simulink model "Model_IPS1"  (R2016a)
settings: Solver=ode45  StartTime=0.0  StopTime=1.5
values from neighbouring files (symbols this model uses):
  Imrn = 7.4    [parametriAM.m]
  In = 12.7    [parametriAM.m]
  Ismax = In*sqrt(2)    [parametriAM.m]
  J = 0.019    [parametriAM.m]
  Lm = 0.0493    [parametriAM.m]
  Lr = 0.05315    [parametriAM.m]
  Ls = 0.05315    [parametriAM.m]
  Ls_oc = Ls    (= 0.05315)    [parametriAM.m]
  Lst = sigma*Ls    (= 0.00742111947319)    [parametriAM.m]
  pp = 3    [parametriAM.m]
  Rs = 0.594    [parametriAM.m]
  Rs_oc = Rs    (= 0.594)    [parametriAM.m]
  sigma = 1 - 1/((1+sigmaR)*(1+sigmaS))    (= 0.13962595434)    [parametriAM.m]
  sigma_oc = 1 - 1/((1+sigmaR_oc)*(1+sigmaS_oc))    (= 0.13962595434)    [parametriAM.m]
  Tr = Lr/Rr    (= 0.0771407837446)    [parametriAM.m]
  Udc = Un*sqrt(2)    [parametriAM.m]
  Un = 216    [parametriAM.m]
  Usmax = Udc    [parametriAM.m]
libraries: simulink x6
settings Model: Creator=Vaje  LastModifiedBy=Mitja1

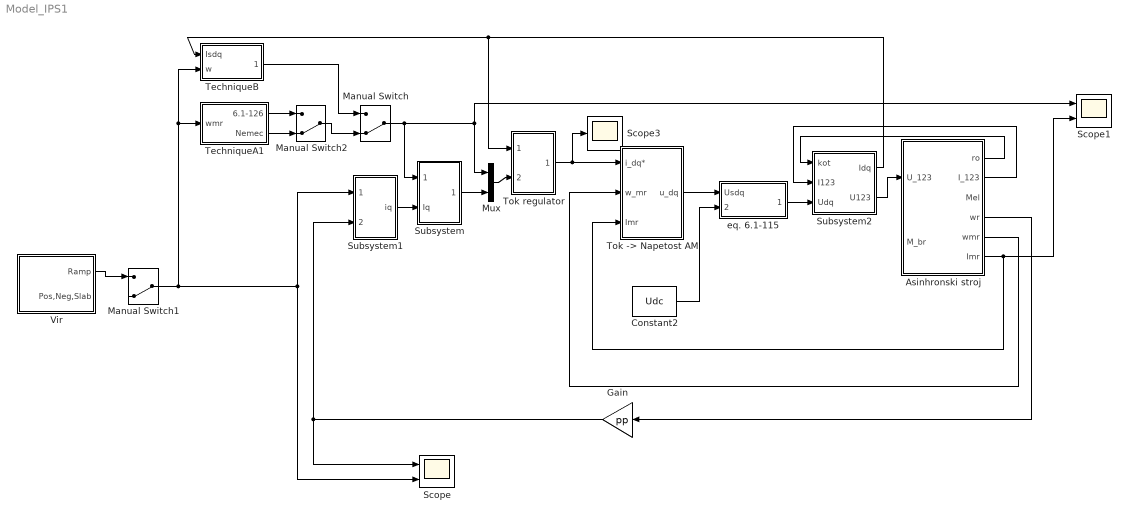
== system Model_IPS1 ==
  Asinhronski stroj : Subsystem  InitFcn=parametriAM
  Constant2 : Constant  Value=Udc
  Gain : Gain  Gain=pp
  Manual Switch : ManualSwitch  CurrentSetting=0
  Manual Switch1 : ManualSwitch  CurrentSetting=0
  Manual Switch2 : ManualSwitch  CurrentSetting=0
  Mux : Mux  Inputs=2
  Scope : Scope  NumInputPorts=2
  Scope1 : Scope  NumInputPorts=2
  Scope3 : Scope
  Subsystem : Subsystem
  Subsystem1 : Subsystem
  Subsystem2 : Subsystem
  TechniqueA1 : Subsystem
  TechniqueB : Subsystem
  "Tok -> Napetost AM" : Subsystem
  Tok regulator : Subsystem
  Vir : Subsystem
  eq. 6.1-115 : Subsystem
  wires:
  Constant2/1 -> eq. 6.1-115/2(Usmax)
  "Tok -> Napetost AM"/1(u_dq) -> eq. 6.1-115/1(Usdq)
  Asinhronski stroj/6(Imr) -> Scope1/2, "Tok -> Napetost AM"/3(Imr)
  Asinhronski stroj/5(wmr) -> "Tok -> Napetost AM"/2(w_mr)
  Tok regulator/1(Idq) -> Scope3/1, "Tok -> Napetost AM"/1(i_dq*)
  Gain/1 -> Scope/1, Subsystem1/2(wfdb)
  Subsystem1/1(iq) -> Subsystem/2(Iq)
  Asinhronski stroj/4(wr) -> Gain/1
  Manual Switch/1 -> Subsystem/1(Idref), Mux/1, Scope1/1
  Manual Switch1/1 -> TechniqueB/2(w), TechniqueA1/1(wmr), Subsystem1/1(wref), Scope/2
  Subsystem/1(Iqlim) -> Mux/2
  TechniqueA1/1(6.1-126) -> Manual Switch2/1
  TechniqueA1/2(Nemec) -> Manual Switch2/2
  Vir/1(Ramp) -> Manual Switch1/1
  Subsystem2/1(Idq) -> Tok regulator/1(Idqdej), TechniqueB/1(Isdq)
  Asinhronski stroj/1(ro) -> Subsystem2/1(kot)
  Asinhronski stroj/2(I_123) -> Subsystem2/2(I123)
  eq. 6.1-115/1(Usdqlim) -> Subsystem2/3(Udq)
  Subsystem2/2(U123) -> Asinhronski stroj/1(U_123)
  TechniqueB/1(6.1-135) -> Manual Switch/1
  Manual Switch2/1 -> Manual Switch/2
  Mux/1 -> Tok regulator/2(Idqref)

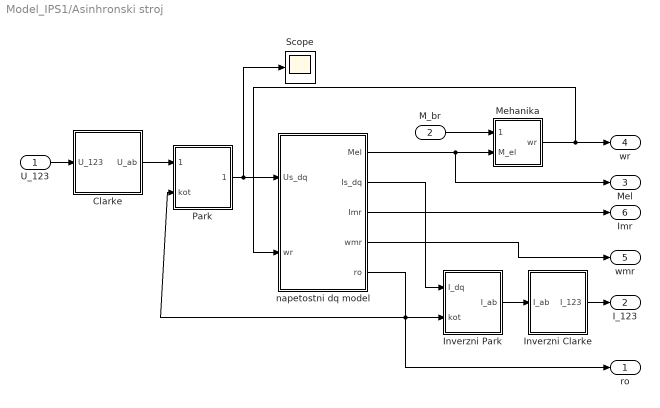
== system Model_IPS1/Asinhronski stroj ==
  U_123 : Inport
  M_br : Inport  Port=2
  Clarke : Subsystem
  Inverzni Clarke : Subsystem
  Inverzni Park : Subsystem
  Mehanika : Subsystem
  Park : Subsystem
  Scope : Scope
  napetostni dq model : Subsystem
  ro : Outport
  I_123 : Outport  Port=2
  Mel : Outport  Port=3
  wr : Outport  Port=4
  wmr : Outport  Port=5
  Imr : Outport  Port=6
  wires:
  Inverzni Park/1(I_ab) -> Inverzni Clarke/1(I_ab)
  Clarke/1(U_ab) -> Park/1(U_ab)
  Mehanika/1(wr) -> napetostni dq model/2(wr), wr/1
  M_br/1 -> Mehanika/1(M_br)
  napetostni dq model/1(Mel) -> Mel/1, Mehanika/2(M_el)
  Inverzni Clarke/1(I_123) -> I_123/1
  napetostni dq model/4(wmr) -> wmr/1
  napetostni dq model/3(Imr) -> Imr/1
  U_123/1 -> Clarke/1(U_123)
  napetostni dq model/2(Is_dq) -> Inverzni Park/1(I_dq)
  napetostni dq model/5(ro) -> ro/1, Park/2(kot), Inverzni Park/2(kot)
  Park/1(U_dq) -> Scope/1, napetostni dq model/1(Us_dq)

== system Model_IPS1/Subsystem ==
  Idref : Inport
  Iq : Inport  Port=2
  Add1 : Sum  Inputs=-+
  Constant : Constant  Value=In*sqrt(2)
  Gain1 : Gain  Gain=-1
  Product : Product
  Product1 : Product
  Saturation Dynamic : simulink/Discontinuities/Saturation Dynamic  OutMin=[]  OutMax=[]  OutDataTypeStr=Inherit: Same as second input  OutDataType=fixdt(1, 16)  OutScaling=2^-10  DoSatur=off
  Sqrt : Sqrt  SaturateOnIntegerOverflow=on
  Iqlim : Outport
  wires:
  Constant/1 -> Product/1, Product/2
  Sqrt/1 -> Gain1/1, Saturation Dynamic/1
  Product1/1 -> Add1/1
  Gain1/1 -> Saturation Dynamic/3
  Add1/1 -> Sqrt/1
  Iq/1 -> Saturation Dynamic/2
  Idref/1 -> Product1/2, Product1/1
  Saturation Dynamic/1 -> Iqlim/1
  Product/1 -> Add1/2

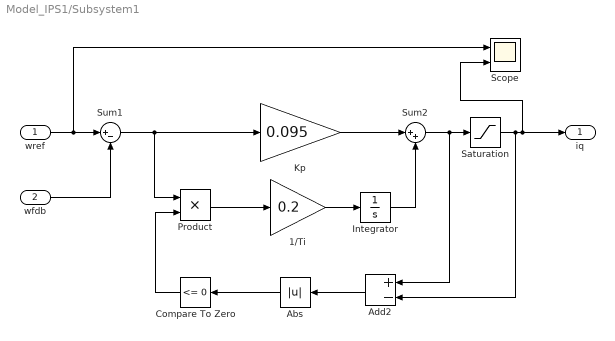
== system Model_IPS1/Subsystem1 ==
  wref : Inport
  wfdb : Inport  Port=2
  1/Ti : Gain  Gain=0.2  SaturateOnIntegerOverflow=on  OutDataTypeStr=Inherit: Same as input  ParamDataTypeStr=Inherit: Same as input
  Abs : Abs
  Add2 : Sum  Inputs=+-
  Compare To Zero : simulink/Logic and Bit Operations/Compare To Zero  relop=<=  OutDataTypeStr=boolean
  Integrator : Integrator
  Kp : Gain  Gain=0.095  SaturateOnIntegerOverflow=on  OutDataTypeStr=Inherit: Same as input  ParamDataTypeStr=Inherit: Same as input
  Product : Product
  Saturation : Saturate  UpperLimit=In*3  LowerLimit=-3*In
  Scope : Scope  NumInputPorts=2
  Sum1 : Sum  Inputs=|+-
  Sum2 : Sum  Inputs=|++
  iq : Outport
  wires:
  1/Ti/1 -> Integrator/1
  Sum1/1 -> Product/1, Kp/1
  Integrator/1 -> Sum2/2
  Sum2/1 -> Add2/1, Saturation/1
  Add2/1 -> Abs/1
  Saturation/1 -> Add2/2, Scope/2, iq/1
  Abs/1 -> Compare To Zero/1
  Kp/1 -> Sum2/1
  Compare To Zero/1 -> Product/2
  Product/1 -> 1/Ti/1
  wref/1 -> Scope/1, Sum1/1
  wfdb/1 -> Sum1/2

== system Model_IPS1/Subsystem2 ==
  kot : Inport
  I123 : Inport  Port=2
  Udq : Inport  Port=3
  Clarke : Subsystem
  Inverzni Clarke : Subsystem
  Inverzni Park : Subsystem
  Park : Subsystem
  Idq : Outport
  U123 : Outport  Port=2
  wires:
  Inverzni Clarke/1(U_123) -> U123/1
  Park/1(I_dq) -> Idq/1
  kot/1 -> Park/2(kot), Inverzni Park/1(kot)
  Clarke/1(I_ab) -> Park/1(I_ab)
  Inverzni Park/1(U_ab) -> Inverzni Clarke/1(U_ab)
  Udq/1 -> Inverzni Park/2(U_dq)
  I123/1 -> Clarke/1(I_123)

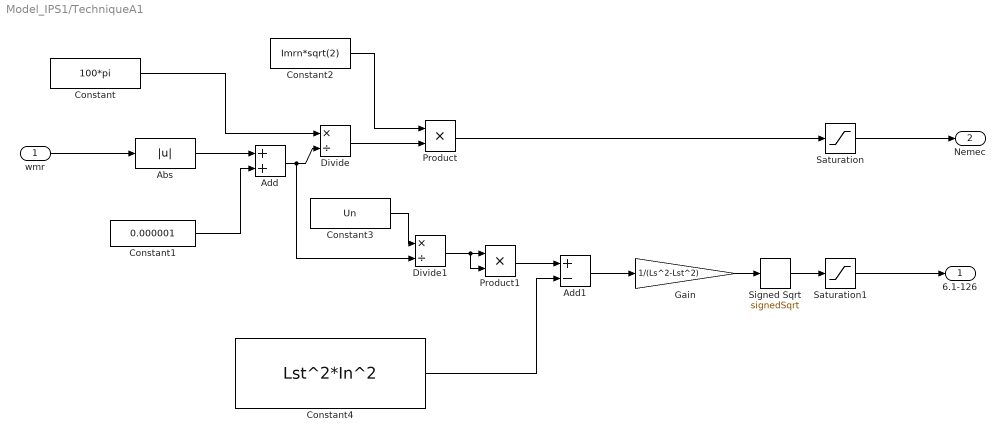
== system Model_IPS1/TechniqueA1 ==
  wmr : Inport
  Abs : Abs
  Add : Sum
  Add1 : Sum  Inputs=+-
  Constant : Constant  Value=100*pi
  Constant1 : Constant  Value=0.000001
  Constant2 : Constant  Value=Imrn*sqrt(2)
  Constant3 : Constant  Value=Un
  Constant4 : Constant  Value=Lst^2*In^2
  Divide : Product  Inputs=*/
  Divide1 : Product  Inputs=*/
  Gain : Gain  Gain=1/(Ls^2-Lst^2)
  Product : Product
  Product1 : Product
  Saturation : Saturate  UpperLimit=+Imrn*sqrt(2)  LowerLimit=0
  Saturation1 : Saturate  UpperLimit=+Imrn*sqrt(2)  LowerLimit=0
  Signed Sqrt : Sqrt  Operator=signedSqrt  SaturateOnIntegerOverflow=on
  6.1-126 : Outport
  Nemec : Outport  Port=2
  wires:
  Constant2/1 -> Product/1
  wmr/1 -> Abs/1
  Divide/1 -> Product/2
  Product/1 -> Saturation/1
  Constant/1 -> Divide/1
  Add/1 -> Divide1/2, Divide/2
  Abs/1 -> Add/1
  Constant1/1 -> Add/2
  Saturation/1 -> Nemec/1
  Constant3/1 -> Divide1/1
  Divide1/1 -> Product1/2, Product1/1
  Product1/1 -> Add1/1
  Constant4/1 -> Add1/2
  Saturation1/1 -> 6.1-126/1
  Add1/1 -> Gain/1
  Gain/1 -> Signed Sqrt/1
  Signed Sqrt/1 -> Saturation1/1

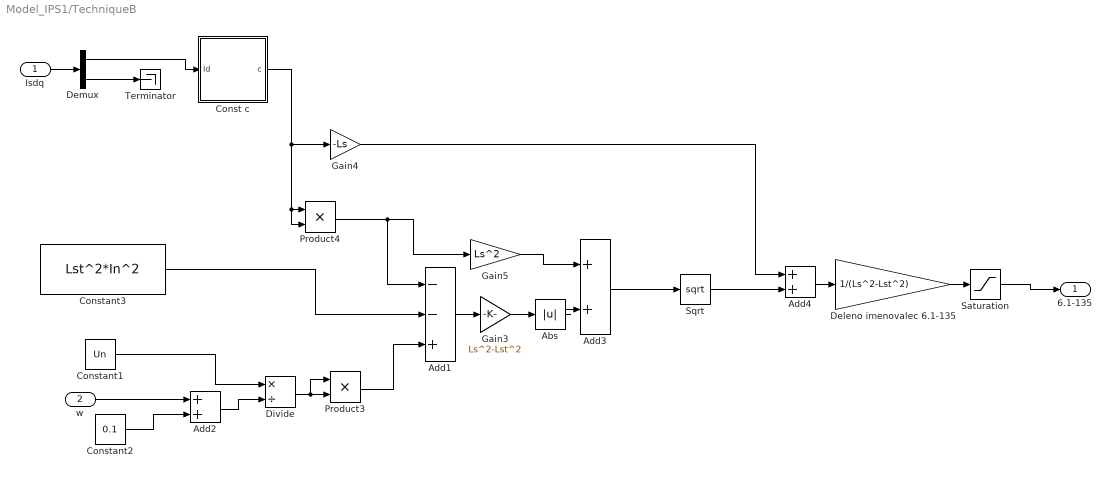
== system Model_IPS1/TechniqueB ==
  Isdq : Inport
  w : Inport  Port=2
  Abs : Abs
  Add1 : Sum  Inputs=--+
  Add2 : Sum
  Add3 : Sum
  Add4 : Sum
  Const c : Subsystem
  Constant1 : Constant  Value=Un
  Constant2 : Constant  Value=0.1
  Constant3 : Constant  Value=Lst^2*In^2
  Deleno imenovalec 6.1-135 : Gain  Gain=1/(Ls^2-Lst^2)
  Demux : Demux  Outputs=2
  Divide : Product  Inputs=*/
  Gain3 : Gain  Gain=Ls^2-Lst^2
  Gain4 : Gain  Gain=-Ls
  Gain5 : Gain  Gain=Ls^2
  Product3 : Product
  Product4 : Product
  Saturation : Saturate  UpperLimit=+Imrn*sqrt(2)  LowerLimit=0
  Sqrt : Sqrt  SaturateOnIntegerOverflow=on
  Terminator : Terminator
  6.1-135 : Outport
  wires:
  Isdq/1 -> Demux/1
  Constant1/1 -> Divide/1
  w/1 -> Add2/1
  Constant2/1 -> Add2/2
  Demux/1 -> Const c/1(Id)
  Demux/2 -> Terminator/1
  Saturation/1 -> 6.1-135/1
  Const c/1(c) -> Product4/2, Product4/1, Gain4/1
  Product4/1 -> Add1/1, Gain5/1
  Gain5/1 -> Add3/1
  Gain4/1 -> Add4/1
  Add4/1 -> Deleno imenovalec 6.1-135/1
  Deleno imenovalec 6.1-135/1 -> Saturation/1
  Add1/1 -> Gain3/1
  Constant3/1 -> Add1/2
  Add2/1 -> Divide/2
  Divide/1 -> Product3/1, Product3/2
  Product3/1 -> Add1/3
  Sqrt/1 -> Add4/2
  Gain3/1 -> Abs/1
  Add3/1 -> Sqrt/1
  Abs/1 -> Add3/2

== system Model_IPS1/Tok -> Napetost AM ==
  i_dq* : Inport
  w_mr : Inport  Port=2
  Imr : Inport  Port=3
  Mux : Mux  Inputs=2
  eq 5.146 : Subsystem
  eq 5.147 : Subsystem
  u_dq : Outport
  wires:
  i_dq*/1 -> eq 5.147/1(I_dq), eq 5.146/1(I_dq)
  Mux/1 -> u_dq/1
  w_mr/1 -> eq 5.147/2(w_mr), eq 5.146/2(w_mr)
  Imr/1 -> eq 5.146/3(Imr), eq 5.147/3(Imr)
  eq 5.147/1(u_q) -> Mux/2
  eq 5.146/1(u_d) -> Mux/1

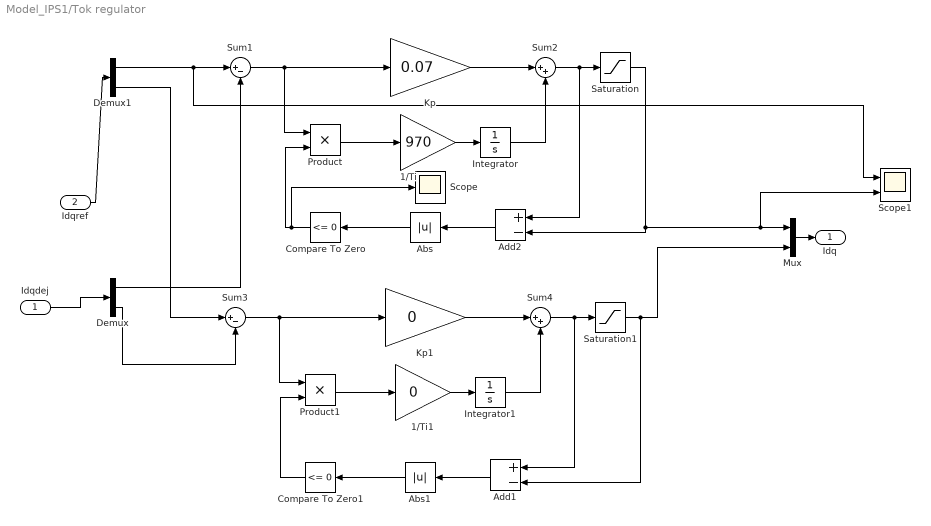
== system Model_IPS1/Tok regulator ==
  Idqdej : Inport
  Idqref : Inport  Port=2
  1/Ti : Gain  Gain=970  SaturateOnIntegerOverflow=on  OutDataTypeStr=Inherit: Same as input  ParamDataTypeStr=Inherit: Same as input
  1/Ti1 : Gain  Gain=0  SaturateOnIntegerOverflow=on  OutDataTypeStr=Inherit: Same as input  ParamDataTypeStr=Inherit: Same as input
  Abs : Abs  ZeroCross=off
  Abs1 : Abs
  Add1 : Sum  Inputs=+-
  Add2 : Sum  Inputs=+-
  Compare To Zero : simulink/Logic and Bit Operations/Compare To Zero  relop=<=  OutDataTypeStr=boolean  ZeroCross=off
  Compare To Zero1 : simulink/Logic and Bit Operations/Compare To Zero  relop=<=  OutDataTypeStr=boolean
  Demux : Demux  Outputs=2
  Demux1 : Demux  Outputs=2
  Integrator : Integrator
  Integrator1 : Integrator
  Kp : Gain  Gain=0.07  SaturateOnIntegerOverflow=on  OutDataTypeStr=Inherit: Same as input  ParamDataTypeStr=Inherit: Same as input
  Kp1 : Gain  Gain=0  SaturateOnIntegerOverflow=on  OutDataTypeStr=Inherit: Same as input  ParamDataTypeStr=Inherit: Same as input
  Mux : Mux  Inputs=2
  Product : Product
  Product1 : Product
  Saturation : Saturate  UpperLimit=Ismax  LowerLimit=-Ismax  ZeroCross=off
  Saturation1 : Saturate  UpperLimit=3*In  LowerLimit=-3*In
  Scope : Scope
  Scope1 : Scope  NumInputPorts=2
  Sum1 : Sum  Inputs=|+-
  Sum2 : Sum  Inputs=|++
  Sum3 : Sum  Inputs=|+-
  Sum4 : Sum  Inputs=|++
  Idq : Outport
  wires:
  Abs1/1 -> Compare To Zero1/1
  Add1/1 -> Abs1/1
  Compare To Zero1/1 -> Product1/2
  Product1/1 -> 1/Ti1/1
  Integrator1/1 -> Sum4/2
  Sum4/1 -> Saturation1/1, Add1/1
  Saturation1/1 -> Mux/2, Add1/2
  Kp1/1 -> Sum4/1
  1/Ti1/1 -> Integrator1/1
  Sum3/1 -> Kp1/1, Product1/1
  Demux1/2 -> Sum3/1
  Idqref/1 -> Demux1/1
  Mux/1 -> Idq/1
  Sum1/1 -> Product/1, Kp/1
  Integrator/1 -> Sum2/2
  Saturation/1 -> Scope1/2, Mux/1, Add2/2
  Kp/1 -> Sum2/1
  Demux1/1 -> Scope1/1, Sum1/1
  1/Ti/1 -> Integrator/1
  Add2/1 -> Abs/1
  Abs/1 -> Compare To Zero/1
  Compare To Zero/1 -> Scope/1, Product/2
  Sum2/1 -> Add2/1, Saturation/1
  Product/1 -> 1/Ti/1
  Idqdej/1 -> Demux/1
  Demux/2 -> Sum3/2
  Demux/1 -> Sum1/2

== system Model_IPS1/Vir ==
  Add1 : Sum  Inputs=++++
  Rampa : simulink/Sources/Ramp  slope=200*pi  start=0  X0=0
  Step : Step  After=100*pi  SampleTime=0
  Step1 : Step  Time=3  After=100*pi  SampleTime=0
  Step2 : Step  Time=5  After=-300*pi  SampleTime=0
  Step3 : Step  Time=7  After=-100*pi  SampleTime=0
  Ramp : Outport
  Pos,Neg,Slab : Outport  Port=2
  wires:
  Add1/1 -> Pos,Neg,Slab/1
  Step1/1 -> Add1/2
  Step2/1 -> Add1/3
  Step/1 -> Add1/1
  Rampa/1 -> Ramp/1
  Step3/1 -> Add1/4

== system Model_IPS1/eq. 6.1-115 ==
  Usdq : Inport
  Usmax : Inport  Port=2
  Demux : Demux  Outputs=2
  Mux1 : Mux  Inputs=2
  eq. 6.1-120 : Subsystem
  Usdqlim : Outport
  wires:
  Mux1/1 -> Usdqlim/1
  Usdq/1 -> Demux/1
  Usmax/1 -> eq. 6.1-120/3(Usmax)
  Demux/2 -> eq. 6.1-120/2(Usq)
  Demux/1 -> eq. 6.1-120/1(Usd), Mux1/1
  eq. 6.1-120/1(Usqlim) -> Mux1/2

== system Model_IPS1/Asinhronski stroj/Clarke ==
  U_123 : Inport
  ABC_ab1 : Subsystem
  Demux : Demux  Outputs=3
  Mux : Mux  Inputs=2
  U_ab : Outport
  wires:
  Mux/1 -> U_ab/1
  ABC_ab1/2(beta) -> Mux/2
  ABC_ab1/1(alfa) -> Mux/1
  Demux/3 -> ABC_ab1/3(C)
  Demux/2 -> ABC_ab1/2(B)
  Demux/1 -> ABC_ab1/1(A)
  U_123/1 -> Demux/1

== system Model_IPS1/Asinhronski stroj/Inverzni Clarke ==
  I_ab : Inport
  Demux : Demux  Outputs=2
  Mux : Mux  Inputs=3
  ab_ABC : Subsystem
  I_123 : Outport
  wires:
  ab_ABC/3(C) -> Mux/3
  ab_ABC/2(B) -> Mux/2
  ab_ABC/1(A) -> Mux/1
  Demux/2 -> ab_ABC/2(beta)
  Demux/1 -> ab_ABC/1(alfa)
  I_ab/1 -> Demux/1
  Mux/1 -> I_123/1

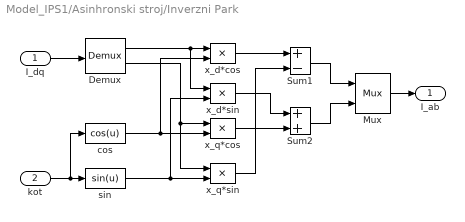
== system Model_IPS1/Asinhronski stroj/Inverzni Park ==
  I_dq : Inport
  kot : Inport  Port=2
  Demux : Demux  Outputs=2
  Mux : Mux  Inputs=2
  "Sum1 " : Sum  Inputs=+-  SaturateOnIntegerOverflow=on  InputSameDT=on  OutDataTypeStr=Inherit: Same as first input
  Sum2 : Sum  SaturateOnIntegerOverflow=on  InputSameDT=on  OutDataTypeStr=Inherit: Same as first input
  cos : Fcn  Expr=cos(u)
  sin : Fcn  Expr=sin(u)
  x_d*cos : Product  SaturateOnIntegerOverflow=on  RndMeth=Zero  InputSameDT=on  OutDataTypeStr=Inherit: Same as first input
  x_d*sin : Product  SaturateOnIntegerOverflow=on  RndMeth=Zero  InputSameDT=on  OutDataTypeStr=Inherit: Same as first input
  x_q*cos : Product  SaturateOnIntegerOverflow=on  RndMeth=Zero  InputSameDT=on  OutDataTypeStr=Inherit: Same as first input
  "x_q*sin " : Product  SaturateOnIntegerOverflow=on  RndMeth=Zero  InputSameDT=on  OutDataTypeStr=Inherit: Same as first input
  I_ab : Outport
  wires:
  Mux/1 -> I_ab/1
  I_dq/1 -> Demux/1
  Demux/1 -> x_d*sin/1, x_d*cos/1
  Demux/2 -> "x_q*sin "/1, x_q*cos/1
  cos/1 -> x_q*cos/2, x_d*cos/2
  sin/1 -> "x_q*sin "/2, x_d*sin/2
  x_d*cos/1 -> "Sum1 "/1
  "x_q*sin "/1 -> "Sum1 "/2
  x_q*cos/1 -> Sum2/2
  x_d*sin/1 -> Sum2/1
  "Sum1 "/1 -> Mux/1
  Sum2/1 -> Mux/2
  kot/1 -> cos/1, sin/1

== system Model_IPS1/Asinhronski stroj/Mehanika ==
  M_br : Inport
  M_el : Inport  Port=2
  Sum : Sum  Inputs=+-
  eq 2.19 : Subsystem
  wr : Outport
  wires:
  M_br/1 -> Sum/2
  Sum/1 -> eq 2.19/1(M)
  M_el/1 -> Sum/1
  eq 2.19/1(wr) -> wr/1

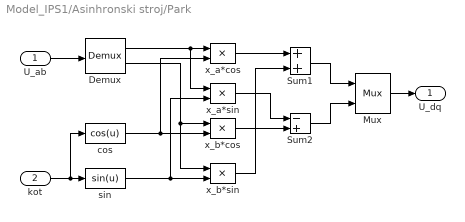
== system Model_IPS1/Asinhronski stroj/Park ==
  U_ab : Inport
  kot : Inport  Port=2
  Demux : Demux  Outputs=2
  Mux : Mux  Inputs=2
  "Sum1 " : Sum  SaturateOnIntegerOverflow=on  InputSameDT=on  OutDataTypeStr=Inherit: Same as first input
  Sum2 : Sum  Inputs=-+  SaturateOnIntegerOverflow=on  InputSameDT=on  OutDataTypeStr=Inherit: Same as first input
  cos : Fcn  Expr=cos(u)
  sin : Fcn  Expr=sin(u)
  x_a*cos : Product  SaturateOnIntegerOverflow=on  RndMeth=Zero  InputSameDT=on  OutDataTypeStr=Inherit: Same as first input
  x_a*sin : Product  SaturateOnIntegerOverflow=on  RndMeth=Zero  InputSameDT=on  OutDataTypeStr=Inherit: Same as first input
  x_b*cos : Product  SaturateOnIntegerOverflow=on  RndMeth=Zero  InputSameDT=on  OutDataTypeStr=Inherit: Same as first input
  "x_b*sin " : Product  SaturateOnIntegerOverflow=on  RndMeth=Zero  InputSameDT=on  OutDataTypeStr=Inherit: Same as first input
  U_dq : Outport
  wires:
  Mux/1 -> U_dq/1
  U_ab/1 -> Demux/1
  Demux/1 -> x_a*sin/1, x_a*cos/1
  Demux/2 -> "x_b*sin "/1, x_b*cos/1
  cos/1 -> x_b*cos/2, x_a*cos/2
  sin/1 -> "x_b*sin "/2, x_a*sin/2
  x_a*cos/1 -> "Sum1 "/1
  "x_b*sin "/1 -> "Sum1 "/2
  x_b*cos/1 -> Sum2/2
  x_a*sin/1 -> Sum2/1
  "Sum1 "/1 -> Mux/1
  Sum2/1 -> Mux/2
  kot/1 -> cos/1, sin/1

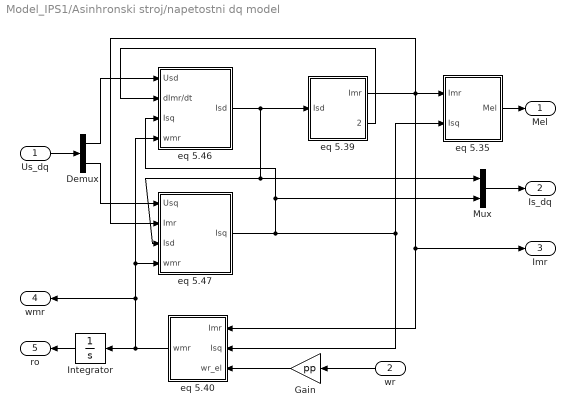
== system Model_IPS1/Asinhronski stroj/napetostni dq model ==
  Us_dq : Inport
  wr : Inport  Port=2
  Demux : Demux  Outputs=2
  Gain : Gain  Gain=pp
  Integrator : Integrator
  Mux : Mux  Inputs=2
  eq 5.35 : Subsystem
  eq 5.39 : Subsystem
  eq 5.40 : Subsystem
  eq 5.46 : Subsystem
  eq 5.47 : Subsystem
  Mel : Outport
  Is_dq : Outport  Port=2
  Imr : Outport  Port=3
  wmr : Outport  Port=4
  ro : Outport  Port=5
  wires:
  Gain/1 -> eq 5.40/3(wr_el)
  Mux/1 -> Is_dq/1
  Demux/2 -> eq 5.47/1(Usq)
  Demux/1 -> eq 5.46/1(Usd)
  Us_dq/1 -> Demux/1
  wr/1 -> Gain/1
  Integrator/1 -> ro/1
  eq 5.35/1(Mel) -> Mel/1
  eq 5.40/1(wmr) -> Integrator/1, wmr/1, eq 5.46/4(wmr), eq 5.47/4(wmr)
  eq 5.47/1(Isq) -> Mux/2, eq 5.46/3(Isq), eq 5.40/2(Isq), eq 5.35/2(Isq)
  eq 5.39/1(Imr) -> eq 5.47/2(Imr), Imr/1, eq 5.40/1(Imr), eq 5.35/1(Imr)
  eq 5.39/2(dImr/dt) -> eq 5.46/2(dImr/dt)
  eq 5.46/1(Isd) -> Mux/1, eq 5.47/3(Isd), eq 5.39/1(Isd)

== system Model_IPS1/Subsystem2/Clarke ==
  I_123 : Inport
  ABC_ab1 : Subsystem
  Demux : Demux  Outputs=3
  Mux : Mux  Inputs=2
  I_ab : Outport
  wires:
  Mux/1 -> I_ab/1
  ABC_ab1/2(beta) -> Mux/2
  ABC_ab1/1(alfa) -> Mux/1
  Demux/3 -> ABC_ab1/3(C)
  Demux/2 -> ABC_ab1/2(B)
  Demux/1 -> ABC_ab1/1(A)
  I_123/1 -> Demux/1

== system Model_IPS1/Subsystem2/Inverzni Clarke ==
  U_ab : Inport
  Demux : Demux  Outputs=2
  Mux : Mux  Inputs=3
  ab_ABC : Subsystem
  U_123 : Outport
  wires:
  ab_ABC/3(C) -> Mux/3
  ab_ABC/2(B) -> Mux/2
  ab_ABC/1(A) -> Mux/1
  Demux/2 -> ab_ABC/2(beta)
  Demux/1 -> ab_ABC/1(alfa)
  U_ab/1 -> Demux/1
  Mux/1 -> U_123/1

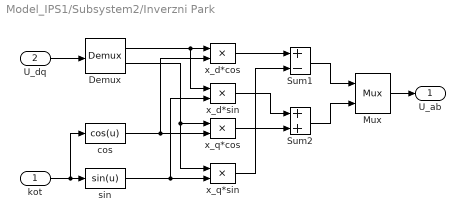
== system Model_IPS1/Subsystem2/Inverzni Park ==
  kot : Inport
  U_dq : Inport  Port=2
  Demux : Demux  Outputs=2
  Mux : Mux  Inputs=2
  "Sum1 " : Sum  Inputs=+-  SaturateOnIntegerOverflow=on  InputSameDT=on  OutDataTypeStr=Inherit: Same as first input
  Sum2 : Sum  SaturateOnIntegerOverflow=on  InputSameDT=on  OutDataTypeStr=Inherit: Same as first input
  cos : Fcn  Expr=cos(u)
  sin : Fcn  Expr=sin(u)
  x_d*cos : Product  SaturateOnIntegerOverflow=on  RndMeth=Zero  InputSameDT=on  OutDataTypeStr=Inherit: Same as first input
  x_d*sin : Product  SaturateOnIntegerOverflow=on  RndMeth=Zero  InputSameDT=on  OutDataTypeStr=Inherit: Same as first input
  x_q*cos : Product  SaturateOnIntegerOverflow=on  RndMeth=Zero  InputSameDT=on  OutDataTypeStr=Inherit: Same as first input
  "x_q*sin " : Product  SaturateOnIntegerOverflow=on  RndMeth=Zero  InputSameDT=on  OutDataTypeStr=Inherit: Same as first input
  U_ab : Outport
  wires:
  Mux/1 -> U_ab/1
  U_dq/1 -> Demux/1
  Demux/1 -> x_d*sin/1, x_d*cos/1
  Demux/2 -> "x_q*sin "/1, x_q*cos/1
  cos/1 -> x_q*cos/2, x_d*cos/2
  sin/1 -> "x_q*sin "/2, x_d*sin/2
  x_d*cos/1 -> "Sum1 "/1
  "x_q*sin "/1 -> "Sum1 "/2
  x_q*cos/1 -> Sum2/2
  x_d*sin/1 -> Sum2/1
  "Sum1 "/1 -> Mux/1
  Sum2/1 -> Mux/2
  kot/1 -> cos/1, sin/1

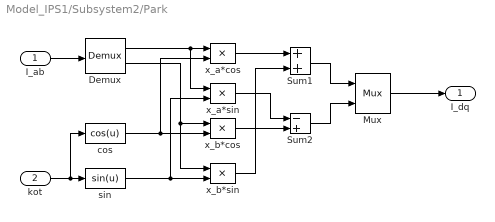
== system Model_IPS1/Subsystem2/Park ==
  I_ab : Inport
  kot : Inport  Port=2
  Demux : Demux  Outputs=2
  Mux : Mux  Inputs=2
  "Sum1 " : Sum  SaturateOnIntegerOverflow=on  InputSameDT=on  OutDataTypeStr=Inherit: Same as first input
  Sum2 : Sum  Inputs=-+  SaturateOnIntegerOverflow=on  InputSameDT=on  OutDataTypeStr=Inherit: Same as first input
  cos : Fcn  Expr=cos(u)
  sin : Fcn  Expr=sin(u)
  x_a*cos : Product  SaturateOnIntegerOverflow=on  RndMeth=Zero  InputSameDT=on  OutDataTypeStr=Inherit: Same as first input
  x_a*sin : Product  SaturateOnIntegerOverflow=on  RndMeth=Zero  InputSameDT=on  OutDataTypeStr=Inherit: Same as first input
  x_b*cos : Product  SaturateOnIntegerOverflow=on  RndMeth=Zero  InputSameDT=on  OutDataTypeStr=Inherit: Same as first input
  "x_b*sin " : Product  SaturateOnIntegerOverflow=on  RndMeth=Zero  InputSameDT=on  OutDataTypeStr=Inherit: Same as first input
  I_dq : Outport
  wires:
  Mux/1 -> I_dq/1
  I_ab/1 -> Demux/1
  Demux/1 -> x_a*sin/1, x_a*cos/1
  Demux/2 -> "x_b*sin "/1, x_b*cos/1
  cos/1 -> x_b*cos/2, x_a*cos/2
  sin/1 -> "x_b*sin "/2, x_a*sin/2
  x_a*cos/1 -> "Sum1 "/1
  "x_b*sin "/1 -> "Sum1 "/2
  x_b*cos/1 -> Sum2/2
  x_a*sin/1 -> Sum2/1
  "Sum1 "/1 -> Mux/1
  Sum2/1 -> Mux/2
  kot/1 -> cos/1, sin/1

== system Model_IPS1/TechniqueB/Const c ==
  Id : Inport
  6.1-131 : TransferFcn  Numerator=[Tr 0]  Denominator=[Tr 1]
  konstanta c : Gain  Gain=Lm^2/Lr
  c : Outport
  wires:
  Id/1 -> 6.1-131/1
  6.1-131/1 -> konstanta c/1
  konstanta c/1 -> c/1

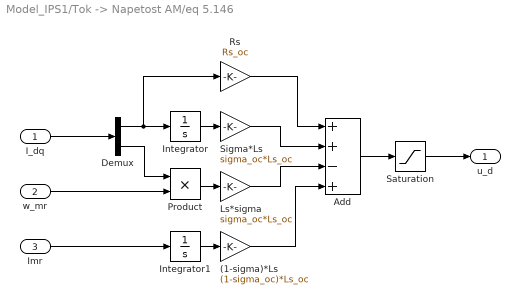
== system Model_IPS1/Tok -> Napetost AM/eq 5.146 ==
  I_dq : Inport
  w_mr : Inport  Port=2
  Imr : Inport  Port=3
  (1-sigma)*Ls : Gain  Gain=(1-sigma_oc)*Ls_oc
  Add : Sum  Inputs=++-+
  Demux : Demux  Outputs=2
  Integrator : Integrator
  Integrator1 : Integrator
  Ls*sigma : Gain  Gain=sigma_oc*Ls_oc
  Product : Product
  Rs : Gain  Gain=Rs_oc
  Saturation : Saturate  UpperLimit=Usmax  LowerLimit=-Usmax
  Sigma*Ls : Gain  Gain=sigma_oc*Ls_oc
  u_d : Outport
  wires:
  w_mr/1 -> Product/2
  Product/1 -> Ls*sigma/1
  Demux/2 -> Product/1
  (1-sigma)*Ls/1 -> Add/4
  Integrator/1 -> Sigma*Ls/1
  Rs/1 -> Add/1
  Sigma*Ls/1 -> Add/2
  Integrator1/1 -> (1-sigma)*Ls/1
  Demux/1 -> Integrator/1, Rs/1
  Ls*sigma/1 -> Add/3
  Add/1 -> Saturation/1
  I_dq/1 -> Demux/1
  Imr/1 -> Integrator1/1
  Saturation/1 -> u_d/1

== system Model_IPS1/Tok -> Napetost AM/eq 5.147 ==
  I_dq : Inport
  w_mr : Inport  Port=2
  Imr : Inport  Port=3
  (1-sigma)*Ls : Gain  Gain=(1-sigma_oc)*Ls_oc
  Add : Sum  Inputs=++++
  Demux : Demux  Outputs=2
  Integrator : Integrator
  Ls*sigma : Gain  Gain=sigma_oc*Ls_oc
  Product : Product
  Product1 : Product
  Rs : Gain  Gain=Rs_oc
  Sigma*Ls : Gain  Gain=sigma_oc*Ls_oc
  u_q : Outport
  wires:
  w_mr/1 -> Product1/1, Product/2
  Product/1 -> Ls*sigma/1
  (1-sigma)*Ls/1 -> Add/4
  Integrator/1 -> Sigma*Ls/1
  Rs/1 -> Add/1
  Sigma*Ls/1 -> Add/2
  Ls*sigma/1 -> Add/3
  Add/1 -> u_q/1
  I_dq/1 -> Demux/1
  Demux/2 -> Integrator/1, Rs/1
  Demux/1 -> Product/1
  Product1/1 -> (1-sigma)*Ls/1
  Imr/1 -> Product1/2

== system Model_IPS1/eq. 6.1-115/eq. 6.1-120 ==
  Usd : Inport
  Usq : Inport  Port=2
  Usmax : Inport  Port=3
  Add : Sum  Inputs=+-
  Gain : Gain  Gain=-1
  Product : Product
  Product1 : Product
  Saturation Dynamic : simulink/Discontinuities/Saturation Dynamic  OutMin=[]  OutMax=[]  OutDataTypeStr=Inherit: Same as second input  OutDataType=fixdt(1, 16)  OutScaling=2^-10  DoSatur=off
  Sqrt : Sqrt  SaturateOnIntegerOverflow=on
  Usqlim : Outport
  wires:
  Usq/1 -> Saturation Dynamic/2
  Saturation Dynamic/1 -> Usqlim/1
  Usd/1 -> Product1/1, Product1/2
  Gain/1 -> Saturation Dynamic/3
  Add/1 -> Sqrt/1
  Product/1 -> Add/1
  Sqrt/1 -> Gain/1, Saturation Dynamic/1
  Product1/1 -> Add/2
  Usmax/1 -> Product/1, Product/2

== system Model_IPS1/Asinhronski stroj/Clarke/ABC_ab1 ==
  A : Inport
  B : Inport  Port=2
  C : Inport  Port=3
  Gain1 : Gain  Gain=2
  Gain2 : Gain
  Gain24 : Gain  Gain=sqrt(3)/3
  Sum11 : Sum
  Terminator : Terminator
  alfa : Outport
  beta : Outport  Port=2
  wires:
  C/1 -> Terminator/1
  Gain1/1 -> Sum11/2
  B/1 -> Gain1/1
  Gain24/1 -> beta/1
  Gain2/1 -> alfa/1
  Sum11/1 -> Gain24/1
  A/1 -> Sum11/1, Gain2/1

== system Model_IPS1/Asinhronski stroj/Inverzni Clarke/ab_ABC ==
  alfa : Inport
  beta : Inport  Port=2
  Gain1 : Gain
  Gain2 : Gain  Gain=-0.5
  Gain25 : Gain  Gain=sqrt(3)/2
  Gain3 : Gain  Gain=sqrt(3)/2
  Gain4 : Gain  Gain=0.5
  Sum10 : Sum
  Sum11 : Sum  Inputs=--
  A : Outport
  B : Outport  Port=2
  C : Outport  Port=3
  wires:
  Gain3/1 -> Sum11/2
  beta/1 -> Gain25/1, Gain3/1
  Gain4/1 -> Sum11/1
  Gain25/1 -> Sum10/2
  Gain2/1 -> Sum10/1
  alfa/1 -> Gain1/1, Gain2/1, Gain4/1
  Gain1/1 -> A/1
  Sum10/1 -> B/1
  Sum11/1 -> C/1

== system Model_IPS1/Asinhronski stroj/Mehanika/eq 2.19 ==
  M : Inport
  Gain1 : Gain  Gain=1/J
  Integrator : Integrator
  wr : Outport
  wires:
  Integrator/1 -> wr/1
  M/1 -> Gain1/1
  Gain1/1 -> Integrator/1

== system Model_IPS1/Asinhronski stroj/napetostni dq model/eq 5.35 ==
  Imr : Inport
  Isq : Inport  Port=2
  Gain : Gain  Gain=3*pp/2
  Gain2 : Gain  Gain=Lm*Lm/Lr
  Product : Product  RndMeth=Zero
  Mel : Outport
  wires:
  Gain/1 -> Gain2/1
  Gain2/1 -> Mel/1
  Product/1 -> Gain/1
  Isq/1 -> Product/2
  Imr/1 -> Product/1

== system Model_IPS1/Asinhronski stroj/napetostni dq model/eq 5.39 ==
  Isd : Inport
  Gain : Gain  Gain=1/Tr
  Integrator : Integrator  InitialCondition=1e-3
  Sum : Sum  Inputs=|+-
  Imr : Outport
  dImr/dt : Outport  Port=2
  wires:
  Gain/1 -> dImr/dt/1, Integrator/1
  Sum/1 -> Gain/1
  Integrator/1 -> Sum/2, Imr/1
  Isd/1 -> Sum/1

== system Model_IPS1/Asinhronski stroj/napetostni dq model/eq 5.40 ==
  Imr : Inport
  Isq : Inport  Port=2
  wr_el : Inport  Port=3
  Divide : Product  Inputs=*/
  Gain2 : Gain  Gain=Tr
  Saturation : Saturate  UpperLimit=2*pi*50  LowerLimit=-2*pi*50
  Sum : Sum  Inputs=|++
  wmr : Outport
  wires:
  Saturation/1 -> Sum/1
  Sum/1 -> wmr/1
  wr_el/1 -> Sum/2
  Divide/1 -> Saturation/1  "ws"
  Gain2/1 -> Divide/2
  Imr/1 -> Gain2/1
  Isq/1 -> Divide/1

== system Model_IPS1/Asinhronski stroj/napetostni dq model/eq 5.46 ==
  Usd : Inport
  dImr/dt : Inport  Port=2
  Isq : Inport  Port=3
  wmr : Inport  Port=4
  Gain : Gain  Gain=1/(sigma*Ls)
  Gain1 : Gain  Gain=Rs
  Gain2 : Gain  Gain=(1-sigma)*Ls
  Gain3 : Gain  Gain=sigma*Ls
  Integrator : Integrator
  Product : Product  RndMeth=Zero
  Sum : Sum  Inputs=+--+
  Isd : Outport
  wires:
  Gain3/1 -> Sum/4
  Product/1 -> Gain3/1
  Isq/1 -> Product/1
  wmr/1 -> Product/2
  Gain2/1 -> Sum/3
  dImr/dt/1 -> Gain2/1
  Gain1/1 -> Sum/2
  Usd/1 -> Sum/1
  Sum/1 -> Gain/1
  Gain/1 -> Integrator/1
  Integrator/1 -> Gain1/1, Isd/1

== system Model_IPS1/Asinhronski stroj/napetostni dq model/eq 5.47 ==
  Usq : Inport
  Imr : Inport  Port=2
  Isd : Inport  Port=3
  wmr : Inport  Port=4
  Gain : Gain  Gain=1/(sigma*Ls)
  Gain1 : Gain  Gain=Rs
  Gain2 : Gain  Gain=(1-sigma)*Ls
  Gain3 : Gain  Gain=sigma*Ls
  Integrator : Integrator
  Product : Product  RndMeth=Zero
  Product1 : Product  RndMeth=Zero
  Sum : Sum  Inputs=+---
  Isq : Outport
  wires:
  Gain3/1 -> Sum/4
  Product1/1 -> Gain3/1
  Isd/1 -> Product1/2
  Gain2/1 -> Sum/3
  Product/1 -> Gain2/1
  wmr/1 -> Product1/1, Product/2
  Imr/1 -> Product/1
  Gain1/1 -> Sum/2
  Usq/1 -> Sum/1
  Sum/1 -> Gain/1
  Gain/1 -> Integrator/1
  Integrator/1 -> Gain1/1, Isq/1

== system Model_IPS1/Subsystem2/Clarke/ABC_ab1 ==
  A : Inport
  B : Inport  Port=2
  C : Inport  Port=3
  Gain1 : Gain  Gain=2
  Gain2 : Gain
  Gain24 : Gain  Gain=sqrt(3)/3
  Sum11 : Sum
  Terminator : Terminator
  alfa : Outport
  beta : Outport  Port=2
  wires:
  C/1 -> Terminator/1
  Gain1/1 -> Sum11/2
  B/1 -> Gain1/1
  Gain24/1 -> beta/1
  Gain2/1 -> alfa/1
  Sum11/1 -> Gain24/1
  A/1 -> Sum11/1, Gain2/1

== system Model_IPS1/Subsystem2/Inverzni Clarke/ab_ABC ==
  alfa : Inport
  beta : Inport  Port=2
  Gain1 : Gain
  Gain2 : Gain  Gain=-0.5
  Gain25 : Gain  Gain=sqrt(3)/2
  Gain3 : Gain  Gain=sqrt(3)/2
  Gain4 : Gain  Gain=0.5
  Sum10 : Sum
  Sum11 : Sum  Inputs=--
  A : Outport
  B : Outport  Port=2
  C : Outport  Port=3
  wires:
  Gain3/1 -> Sum11/2
  beta/1 -> Gain25/1, Gain3/1
  Gain4/1 -> Sum11/1
  Gain25/1 -> Sum10/2
  Gain2/1 -> Sum10/1
  alfa/1 -> Gain1/1, Gain2/1, Gain4/1
  Gain1/1 -> A/1
  Sum10/1 -> B/1
  Sum11/1 -> C/1
